simulink library "motohawk_engine_lib"  (Simulink 6.3)
undefined symbols (not defined in the file or in its folder): cast_val, IndPowerMax, InjSequence, lookup_group, MAF_Sensor_p, motohawk_tex, motohawk_vardec_config_group, motohawk_vardec_path, SampleTime, SparkSequence, SteadyStateECT, txtTitle, WarmUpTimeConst
libraries: MotoHawk_lib x234, motohawk_annotations_lib x22, motohawk_control_primitives_lib x20, motohawk_engine_lib x8, motohawk_control_primitives_lib_new x3
(part 1 of 7)
settings Model: Creator=Blake Suhre  LastModifiedBy=jason_tartt  StrictBusMsg=None

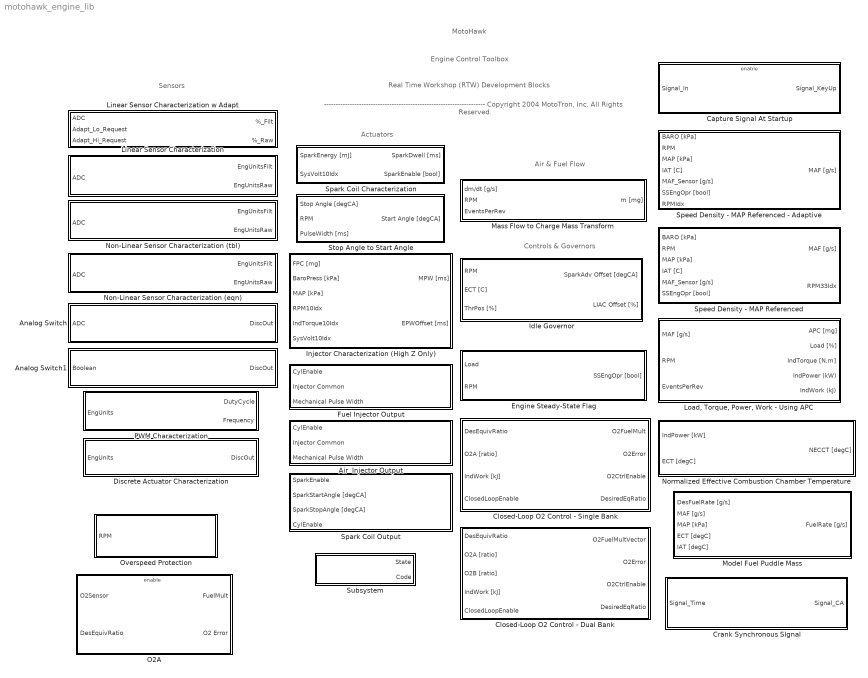
== system motohawk_engine_lib ==
  note: Sensors
  note: MotoHawk
  note: ---------------------------------------------------------------------
      | Copyright 2004 MotoTron, Inc.  All Rights Reserved.
  note: Real Time Workshop (RTW)
      | Development Blocks
  note: Engine Control Toolbox
  note: Actuators
  note: Air & Fuel Flow
  note: Controls & Governors
  Air  Injector Output : Subsystem  mask(Air Injector Hardware Interface){injector=1, offset=InjSequence(1)}
      mask prompts: offset "Angle Offset"
      mask help: Enter the air injector number.
      mask init:
      | lbl = sprintf('TRANSIENT\nAIR INJECTOR %d\n%d DEGREES', injector, offset);
      | 
      | blk = [gcb '/motohawk_injector'];
      | res = sprintf('AINJ%d', injector);
      | set_param(blk, 'text_resource', res);
      mask Display:
      | patch([0 0 1 1], [0 0.075 0.075 0], [230/255 0/255 0/255])
      | patch([0 0 1 1], [0.025 0.05 0.05 0.025], [150/255 0/255 0/255])
      | patch([0 0 1 1], [0 0.025 0.025 0], [0/255 0/255 0/255])
      | 
      | text(0.95, 0.5, lbl, 'horizontalAlignment', 'right');
  Analog Switch : Subsystem  mask{nam='PRNDL_D', prefix='PRNDL_D_', switchpoint=500, polarity=High-True, parent_group=lookup_group(gcb, 'Switches')}
      mask prompts: nam "Name"; switchpoint "Switch Point (ADC)"; parent_group "MotoTune Group"
      mask init:
      | lbl = ['Analog Switch: ' nam ' [bool]'];
      | group = [parent_group ' | ' nam];
      mask StyleString: edit,edit,edit,popup(High-True|Low-True),edit
      mask Display:
      | patch([0 0 1 1], [0 0.075 0.075 0], [230/255 0/255 0/255])
      | patch([0 0 1 1], [0.025 0.05 0.05 0.025], [150/255 0/255 0/255])
      | patch([0 0 1 1], [0 0.025 0.025 0], [0/255 0/255 0/255])
      | 
      | disp(lbl);
  Analog Switch1 : Subsystem  mask{nam='Digital', prefix=Digital_', polarity=High-True, parent_group='Switches'}
      mask prompts: nam "Name"; parent_group "MotoTune Group"
      mask init:
      | lbl = ['Digital Switch: ' nam ' [bool]'];
      | group = [parent_group ' | ' nam];
      mask StyleString: edit,edit,popup(High-True|Low-True),edit
      mask Display:
      | patch([0 0 1 1], [0 0.075 0.075 0], [230/255 0/255 0/255])
      | patch([0 0 1 1], [0.025 0.05 0.05 0.025], [150/255 0/255 0/255])
      | patch([0 0 1 1], [0 0.025 0.025 0], [0/255 0/255 0/255])
      | 
      | disp(lbl);
  Capture Signal At Startup : Subsystem  mask(Capture Signal At Startup){nam='Baro', count=5, units='kPa', grp='Engine Control | Run | Airflow'}
      mask prompts: nam "Signal Name"; count "Number Of Samples To Average"; grp "MotoTune GroupString Name"
      mask init:
      | lbl = sprintf('CAPTURE IN STALL\nAverage of\nfirst %d samples', count);
      mask Display:
      | patch([0 0 1 1], [0 0.075 0.075 0], [230/255 0/255 0/255])
      | patch([0 0 1 1], [0.025 0.05 0.05 0.025], [150/255 0/255 0/255])
      | patch([0 0 1 1], [0 0.025 0.025 0], [0/255 0/255 0/255])
      | 
      | disp(lbl);
  Closed-Loop O2 Control - Dual Bank : Subsystem
      mask Display:
      | patch([0 0 1 1], 0.5*[0 0.075 0.075 0], [230/255 0/255 0/255])
      | patch([0 0 1 1], 0.5*[0.025 0.05 0.05 0.025], [150/255 0/255 0/255])
      | patch([0 0 1 1], 0.5*[0 0.025 0.025 0], [0/255 0/255 0/255])
      | 
      | disp('DUAL BANK \nO2 CONTROL');
  Closed-Loop O2 Control - Single Bank : Subsystem
      mask Display:
      | patch([0 0 1 1], 0.5*[0 0.075 0.075 0], [230/255 0/255 0/255])
      | patch([0 0 1 1], 0.5*[0.025 0.05 0.05 0.025], [150/255 0/255 0/255])
      | patch([0 0 1 1], 0.5*[0 0.025 0.025 0], [0/255 0/255 0/255])
      | 
      | disp('SINGLE BANK \nO2 CONTROL');
  Crank Synchronous SIgnal : Subsystem
      mask Type: Crank Based Sensor Value
      mask Description: This subsystem averages input signal captured at 0 and 360 degrees.
      mask Display:
      | patch([0 0 1 1], [0 0.075 0.075 0], [230/255 0/255 0/255])
      | patch([0 0 1 1], [0.025 0.05 0.05 0.025], [150/255 0/255 0/255])
      | patch([0 0 1 1], [0 0.025 0.025 0], [0/255 0/255 0/255])
      | 
      | disp('CRANK SYNCHRONOUS \nSIGNAL')
  Discrete Actuator Characterization : Subsystem  mask(Discrete Actuator Characterization){prefix='MIL', nam='MIL', units='bool', parent_group='Actuators', polarity=High-True}
      mask prompts: nam "Name"; parent_group "MotoTune Group"
      mask help: Provides the ability to calibrate the polarity of the output digital state before it is applied to the digital output pin.
      mask init:
      | lbl = ['Discrete Characterization:  ' nam ];
      | group = [parent_group ' | ' nam];
      mask StyleString: edit,edit,edit,edit,popup(High-True|Low-True)
      mask Display:
      | patch([0 0 1 1], [0 0.075 0.075 0], [230/255 0/255 0/255])
      | patch([0 0 1 1], [0.025 0.05 0.05 0.025], [150/255 0/255 0/255])
      | patch([0 0 1 1], [0 0.025 0.025 0], [0/255 0/255 0/255])
      | 
      | disp(lbl);
  Engine Steady-State Flag : Subsystem  Description=|  mask(Steady-State Engine Operation){samp_time=SampleTime, group='Engine Control | States | States Config'}
      | /* Name: SSTorqueFilterConst Unit:sec ClassID:VAR StorageID:FLASH Access:RW4+RW3+NA2+NA1 TypeID:UINT2            
      |    Gain:0.001 Min:0.00 Max:65.54 Format:4.2 UpdateID:REMOTE Group:"Engine Control | States" Help:"First-order "  
      |    "filter time constant used to filter torque. This value must be less than SSTorqueTol from unfiltered torque "
      |    "before the steady-state flag can be enabled." VardecSig:6C */                                                
      |                                                                                                                  
      | /* Name: SSRPMFilterConst Unit:sec ClassID:VAR StorageID:FLASH Access:RW4+RW3+NA2+NA1 TypeID:UINT2               
      |    Gain:0.001 Min:0.00 Max:65.54 Format:4.2 UpdateID:REMOTE Group:"Engine Control | States" Help:"First-order "  
      |    "filter time constant used to filter torque. This value must be less than SSRPMTol from unfiltered torque "   
      |    "before the steady-state flag can be enabled." VardecSig:6C */                                                
      |                                                                                                                  
      | /* Name: SSTorqueTol Unit:N.m ClassID:VAR StorageID:FLASH Access:RW4+RW3+NA2+NA1 TypeID:UINT2 Gain:0.001         
      |    Min:0.00 Max:65.54 Format:4.2 UpdateID:REMOTE Group:"Engine Control | States" Help:"Tolerance within which "  
      |    "the difference between filtered and unfiltered torque must lie before the steady-state flag can be "         
      |    "enabled." VardecSig:6C */                                                                                    
      |                                                                                                                  
      | /* Name: SSRPMTol Unit:RPM ClassID:VAR StorageID:FLASH Access:RW4+RW3+NA2+NA1 TypeID:UINT2 Gain:0.01             
      |    Min:0.00 Max:655.35 Format:4.2 UpdateID:REMOTE Group:"Engine Control | States" Help:"Tolerance within which " 
      |    "the difference between filtered and unfiltered RPM must lie before the steady-state flag can be enabled."    
      |    VardecSig:6C */
      mask prompts: samp_time "Sample Time [s]:"; group "MotoTune Group String"
      mask help:
      | This block determines whether or not the engine has achieved steady-state operation. It accomplishes this by applying a first-order low-pass filter to the indicated torque and RPM inputs. The filetrcoeficeints are individually calibratable for each. Once both the filtered torque and RPM values are within the calibratable toleraance of the input values, engine operation is assumed to be steady-state.
      |
      | If 'Sample Time' is -1, then extra code and RAM will be generated to dynamically calculate dt.
      mask Display:
      | patch([0 0 1 1], [0 0.075 0.075 0], [230/255 0/255 0/255])
      | patch([0 0 1 1], [0.025 0.05 0.05 0.025], [150/255 0/255 0/255])
      | patch([0 0 1 1], [0 0.025 0.025 0], [0/255 0/255 0/255])
      | 
      | disp('ENGINE\nSTEADY-STATE\nDETERMINATION')
  Fuel Injector Output : Subsystem  mask(Fuel Injector Hardware Interface){injector=1, offset=InjSequence(1)}
      mask prompts: offset "Angle Offset"
      mask help: Enter the fuel injector number.
      mask init:
      | lbl = sprintf('TRANSIENT\nFUEL INJECTOR %d\n%d DEGREES', injector, offset);
      | 
      | blk = [gcb '/motohawk_injector'];
      | res = sprintf('FINJ%d', injector);
      | set_param(blk, 'text_resource', res);
      mask Display:
      | patch([0 0 1 1], [0 0.075 0.075 0], [230/255 0/255 0/255])
      | patch([0 0 1 1], [0.025 0.05 0.05 0.025], [150/255 0/255 0/255])
      | patch([0 0 1 1], [0 0.025 0.025 0], [0/255 0/255 0/255])
      | 
      | text(0.95, 0.5, lbl, 'horizontalAlignment', 'right');
  Idle Governor : Subsystem
      mask Display:
      | patch([0 0 1 1], 0.5*[0 0.075 0.075 0], [230/255 0/255 0/255])
      | patch([0 0 1 1], 0.5*[0.025 0.05 0.05 0.025], [150/255 0/255 0/255])
      | patch([0 0 1 1], 0.5*[0 0.025 0.025 0], [0/255 0/255 0/255])
      | 
      | disp('IDLE GOVERNOR');
  Injector Characterization (High Z Only) : Subsystem  Description=|
      | /* Name: InjGain Unit:ms/mg ClassID:VAR StorageID:FLASH Access:RW4+RW3+NA2+NA1 TypeID:UINT2 Gain:0.0001       
      |    Min:0.0000 Max:6.5500 Format:5.4 UpdateID:REMOTE Group:"Actuators | Injectors | Config" Help:"Gain valued "
      |    "used in the linear transformation of FPC to mechanical pulsewidth." VardecSig:6C */                       
      |                                                                                                               
      | /* Name: InjOfst Unit:ms ClassID:VAR StorageID:FLASH Access:RW4+RW3+NA2+NA1 TypeID:SINT2 Gain:0.0001          
      |    Min:-3.2768 Max:3.2767 Format:5.4 UpdateID:REMOTE Group:"Actuators | Injectors | Config" Help:"Offset "    
      |    "valued used in the linear transformation of FPC to mechanical pulsewidth." VardecSig:6C */                
      |                                                                                                               
      | /* Name: SysVolt10IdxArr Unit:volt ClassID:ORDARR StorageID:FLASH Access:RW4+RW3+NA2+NA1 TypeID:UINT1         
      |    Gain:0.1 Min:0.00 Max:25.50 Format:4.2 UpdateID:REMOTE OrdLen:10 Group:"Global Index Arrays | Voltage"     
      |    Help:"Ten breakpoint system voltage index array." VardecSig:6C */                                          
      |                                                                                                               
      | /* Name: InjTurnOnTbl Unit:ms ClassID:TBL StorageID:FLASH Access:RW4+RW3+NA2+NA1 TypeID:UINT2 Gain:0.001      
      |    Min:0.0000 Max:65.5350 Format:5.4 UpdateID:REMOTE OrdArr:SysVolt10IdxArr Group:"Actuators | Injectors"     
      |    Help:"Injector turn on time as a function of system voltage." VardecSig:6C */                              
      |                                                                                                               
      | /* Name: InjDeltaPress10IdxArr Unit:kPa ClassID:ORDARR StorageID:FLASH Access:RW4+RW3+NA2+NA1 TypeID:UINT2    
      |    Gain:0.1 Min:0.0 Max:6553.0 Format:5.1 UpdateID:REMOTE OrdLen:10 Group:"Actuators | Injectors" Help:"Ten " 
      |    "breakpoint fuel delta pressure index array." VardecSig:6C */                                              
      |                                                                                                               
      | /* Name: FueldPCompTbl Unit:kPa ClassID:TBL StorageID:FLASH Access:RW4+RW3+NA2+NA1 TypeID:UINT2 Gain:0.1      
      |    Min:0.0 Max:6553.0 Format:5.1 UpdateID:REMOTE OrdArr:InjDeltaPress10IdxArr Group:"Actuators | Injectors"   
      |    Help:"Injector delta pressure compensation table." VardecSig:6C */                                         
      |                                                                                                               
      | /* Name: InjTurnOffTbl Unit:ms ClassID:TBL StorageID:FLASH Access:RW4+RW3+NA2+NA1 TypeID:UINT2                
      |    Gain:0.01 Min:0.00 Max:655.00 Format:5.2 UpdateID:REMOTE OrdArr:InjDeltaPress10IdxArr Group:"Actuators | " 
      |    "Injectors" Help:"Injector turn off time table." VardecSig:6C */                                           
      |                                                                                                               
      | /* Name: InjMPW Unit:ms ClassID:VAR StorageID:RAM Access:RO4+RO3+NA2+NA1 TypeID:UINT2 Gain:0.01 Min:0.00      
      |    Max:655.35 Format:5.2 UpdateID:BACKGND Group:"Actuators | Injectors" Help:"Injector mechanical pulse "     
      |    "width." VardecSig:6C */                                                                                   
      |                                                                                                               
      | /* Name: InjEPW Unit:ms ClassID:VAR StorageID:RAM Access:RO4+RO3+NA2+NA1 TypeID:UINT2 Gain:0.01 Min:0.00      
      |    Max:655.35 Format:5.2 UpdateID:BACKGND Group:"Actuators | Injectors" Help:"Injector electrical pulse "     
      |    "width." VardecSig:6C */                                                                                   
      |                                                                                                               
      | /* Name: InjDeltaPress Unit:kPa ClassID:VAR StorageID:RAM Access:RO4+RO3+NA2+NA1 TypeID:UINT2 Gain:0.01       
      |    Min:0.00 Max:655.35 Format:5.2 UpdateID:BACKGND Group:"Actuators | Injectors" Help:"Delta pressure across "
      |    "the injector." VardecSig:6C */                                                                            
      | /* Name: FuelFlowCompMap Unit:mult ClassID:MAP StorageID:RAM Access:RO4+RO3+NA2+NA1 TypeID:UINT2              
      |    Gain:0.0001 Min:0.0000 Max:2.0000 Format:5.4 UpdateID:BACKGND XOrdArr:IndTorque10IdxArr YOrdArr:RPM10IdxArr
      |    Group:"Actuators | Injectors" Help:"Correction for injector fuel flow differences between injector test "  
      |    "bench and engine operating in the conditions. This map should only be calibrated after volumetric "       
      |    "efficiency has been calibrated to a reference airflow measurement device." VardecSig:6C */
      mask Description: Injector characterization block.
      mask Help: Converts the calculated fuel charge mass (FPC) value to the required electrical pulsewidth. Requires gain, offset, turn-on time vs. voltage, turn-off time vs. injector delta pressure and delta pressure pulsewidth compensation. A choice of five different injector delta pressure calculation methods are offered.
      mask Display:
      | patch([0 0 1 1], [0 0.075 0.075 0], [230/255 0/255 0/255])
      | patch([0 0 1 1], [0.025 0.05 0.05 0.025], [150/255 0/255 0/255])
      | patch([0 0 1 1], [0 0.025 0.025 0], [0/255 0/255 0/255])
      | 
      | disp('INJECTOR\nCHRZN.\n(High Z Only)')
  Linear Sensor Characterization : Subsystem  mask(Linear Sensor Characterization){nam='SysVolt', prefix='SysVolt_', units='Volts', inputunits=0, parent_group='Sensors | System Volts', samp_time=SampleTime}
      mask prompts: nam "Name"; units "Output Units"; inputunits "Input Units"; parent_group "MotoTune Group"; samp_time "Sample Time"
      mask help:
      | Converts from A/D Counts to Engineering Units, using a Gain and Offset.
      | Saturates the converted value around Min and Max values, and triggers a Fault when out of range.
      mask init:
      | lbl = ['Linear Sensor: ' nam ' [' units ']'];
      | group = [parent_group ' | ' nam];
      settings: RTWSystemCode=Function  RTWFcnNameOpts=Use subsystem name  RTWFileNameOpts=Use function name
      mask Display:
      | patch([0 0 1 1], [0 0.075 0.075 0], [230/255 0/255 0/255])
      | patch([0 0 1 1], [0.025 0.05 0.05 0.025], [150/255 0/255 0/255])
      | patch([0 0 1 1], [0 0.025 0.025 0], [0/255 0/255 0/255])
      | 
      | disp(lbl);
  Linear Sensor Characterization w Adapt : Subsystem  mask(Potentiometer Characterization with adapting endpoints.){nam='APP1', prefix='APP1', samp_time=.005, parent_group='Sensors | APP'}
      mask prompts: nam "Name"; samp_time "Sample Time"; parent_group "MotoTune Group"
      mask help:
      | This block transforms the input from a potentiometer into a percentage, refering to the percentage of travel within the scale.
      |
      | The endpoints of the scale will adapt based on the values that block sees on the input.
      mask init:
      | lbl = ['Linear Sensor: ' nam ' [%]'];
      | lbl2 = ['With Adaption'];
      | group = [parent_group ' | ' nam];
      | units = '%';
      mask Display:
      | patch([0 0 1 1], [0 0.075 0.075 0], [230/255 0/255 0/255])
      | patch([0 0 1 1], [0.025 0.05 0.05 0.025], [150/255 0/255 0/255])
      | patch([0 0 1 1], [0 0.025 0.025 0], [0/255 0/255 0/255])
      | 
      | 
      | 
      | text(0.6,0.60,lbl,'horizontalAlignment','center');
      | text(0.6,0.30,lbl2,'horizontalAlignment','center');
  "Load, Torque, Power, Work - Using APC" : Subsystem
      mask Display:
      | patch([0 0 1 1], 0.8*[0 0.075 0.075 0], [230/255 0/255 0/255])
      | patch([0 0 1 1], 0.8*[0.025 0.05 0.05 0.025], [150/255 0/255 0/255])
      | patch([0 0 1 1], 0.8*[0 0.025 0.025 0], [0/255 0/255 0/255])
      | 
      | disp('LOAD, TORQUE,\nPOWER, AND WORK\nCOMPUTATION\nUSING APC');
  Mass Flow to Charge Mass Transform : Subsystem
      mask Description: Converts mass flow rate to the equivalent per cylinder charge mass.
      mask Help:
      | Given the mass flow rate [g/s], RPM and the total number of combustion events per crankshaft revolution, this block calculates the equivalent charge mass ingested per cylinder.
      | 
      | Note: as an example, the number of cylinder events per revolution would be 2 for a four cylinder four-stroke engine and 4 for a four-cylinder two-stroke engine.
      mask Display:
      | patch([0 0 1 1], [0 0.075 0.075 0], [230/255 0/255 0/255])
      | patch([0 0 1 1], [0.025 0.05 0.05 0.025], [150/255 0/255 0/255])
      | patch([0 0 1 1], [0 0.025 0.025 0], [0/255 0/255 0/255])
      | 
      | disp('MASS FLOW\nTO CHARGE MASS\nTRANSFORM')
  Model Fuel Puddle Mass : Subsystem  mask{group_cal='Engine Control | Run | Fuel | Transient Fuel', group_dis='Engine Control | Run | Fuel | Transient Fuel'}
      mask prompts: group_cal "MotoTune Calibration Group String"; group_dis "MotoTune Display Group String"
      mask Display:
      | patch([0 0 1 1], 0.5*[0 0.075 0.075 0], [230/255 0/255 0/255])
      | patch([0 0 1 1], 0.5*[0.025 0.05 0.05 0.025], [150/255 0/255 0/255])
      | patch([0 0 1 1], 0.5*[0 0.025 0.025 0], [0/255 0/255 0/255])
      | 
      | disp('TAU-X\nTRANSIENT\nFUELING');
  Non-Linear Sensor Characterization (eqn) : Subsystem  mask(Non-Linear Sensor Characterization (eqn)){nam='MAF_Sensor', prefix='MAF_Sensor_', units='g/s', inputunits=0, parent_group=lookup_group(gcb, 'MAF_Sensor'), numcoef=MAF_Sensor_p, samp_time=SampleTime}
      mask prompts: nam "Name"; units "Output Units"; inputunits "Input Units"; parent_group "MotoTune Group"; numcoef "Number Of Coefficients"; samp_time "Sample Time"
      mask help:
      | Converts from A/D Counts to Engineering Units using a calibration polynomial.
      | Saturates the converted value around Min and Max values and triggers a Fault when out of range.
      mask init:
      | lbl = ['Non-Linear Sensor (eqn): ' nam ' [' units ']'];
      | group = [parent_group ' | ' nam];
      settings: RTWSystemCode=Function  RTWFcnNameOpts=Use subsystem name  RTWFileNameOpts=Use function name
      mask Display:
      | patch([0 0 1 1], [0 0.075 0.075 0], [230/255 0/255 0/255])
      | patch([0 0 1 1], [0.025 0.05 0.05 0.025], [150/255 0/255 0/255])
      | patch([0 0 1 1], [0 0.025 0.025 0], [0/255 0/255 0/255])
      | 
      | disp(lbl);
  Non-Linear Sensor Characterization (tbl) : Subsystem  mask(Non-Linear Sensor Characterization (tbl)){nam='MMA_Current', prefix='MMA_Current_', units='mA', inputunits='ADC', parent_group='Sensors', tblsize=20, samp_time=SampleTime}
      mask prompts: nam "Name"; units "Output Units"; inputunits "Input Units"; parent_group "MotoTune Group"; tblsize "Table Size"; samp_time "Sample Time"
      mask help:
      | Converts from A/D Counts to Engineering Units using a 1-D Table Lookup.
      | Saturates the converted value around Min and Max values and triggers a Fault when out of range.
      mask init:
      | lbl = ['Non-Linear Sensor (tbl): ' nam ' [' units ']'];
      | group = [parent_group ' | ' nam];
      settings: RTWSystemCode=Function  RTWFcnNameOpts=Use subsystem name  RTWFileNameOpts=Use function name
      mask Display:
      | patch([0 0 1 1], [0 0.075 0.075 0], [230/255 0/255 0/255])
      | patch([0 0 1 1], [0.025 0.05 0.05 0.025], [150/255 0/255 0/255])
      | patch([0 0 1 1], [0 0.025 0.025 0], [0/255 0/255 0/255])
      | 
      | disp(lbl);
  Normalized Effective Combustion Chamber Temperature : Subsystem  Description=|  mask(Steady-State Engine Operatio){}
      | /* Name: SSTorqueFilterConst Unit:sec ClassID:VAR StorageID:FLASH Access:RW4+RW3+NA2+NA1 TypeID:UINT2            
      |    Gain:0.001 Min:0.00 Max:65.54 Format:4.2 UpdateID:REMOTE Group:"Engine Control | States" Help:"First-order "  
      |    "filter time constant used to filter torque. This value must be less than SSTorqueTol from unfiltered torque "
      |    "before the steady-state flag can be enabled." VardecSig:6C */                                                
      |                                                                                                                  
      | /* Name: SSRPMFilterConst Unit:sec ClassID:VAR StorageID:FLASH Access:RW4+RW3+NA2+NA1 TypeID:UINT2               
      |    Gain:0.001 Min:0.00 Max:65.54 Format:4.2 UpdateID:REMOTE Group:"Engine Control | States" Help:"First-order "  
      |    "filter time constant used to filter torque. This value must be less than SSRPMTol from unfiltered torque "   
      |    "before the steady-state flag can be enabled." VardecSig:6C */                                                
      |                                                                                                                  
      | /* Name: SSTorqueTol Unit:N.m ClassID:VAR StorageID:FLASH Access:RW4+RW3+NA2+NA1 TypeID:UINT2 Gain:0.001         
      |    Min:0.00 Max:65.54 Format:4.2 UpdateID:REMOTE Group:"Engine Control | States" Help:"Tolerance within which "  
      |    "the difference between filtered and unfiltered torque must lie before the steady-state flag can be "         
      |    "enabled." VardecSig:6C */                                                                                    
      |                                                                                                                  
      | /* Name: SSRPMTol Unit:RPM ClassID:VAR StorageID:FLASH Access:RW4+RW3+NA2+NA1 TypeID:UINT2 Gain:0.01             
      |    Min:0.00 Max:655.35 Format:4.2 UpdateID:REMOTE Group:"Engine Control | States" Help:"Tolerance within which " 
      |    "the difference between filtered and unfiltered RPM must lie before the steady-state flag can be enabled."    
      |    VardecSig:6C */
      mask Display:
      | patch([0 0 1 1], [0 0.075 0.075 0], [230/255 0/255 0/255])
      | patch([0 0 1 1], [0.025 0.05 0.05 0.025], [150/255 0/255 0/255])
      | patch([0 0 1 1], [0 0.025 0.025 0], [0/255 0/255 0/255])
      | 
      | disp('COMBUSTION CHAMBER\nTEMPERATURE');
  O2A : Subsystem  TreatAsAtomicUnit=on  mask(Closed-Loop O2 Control){bank=A, display_group=lookup_group(gcb, 'O2Display'), cal_group=lookup_group(gcb, 'O2BankA')}
      mask prompts: display_group "MotoTune Display Group"; cal_group "MotoTune Calibration Group"
      mask StyleString: popup(A|B),edit,edit
      mask Display:
      | patch([0 0 1 1], 0.5*[0 0.075 0.075 0], [230/255 0/255 0/255])
      | patch([0 0 1 1], 0.5*[0.025 0.05 0.05 0.025], [150/255 0/255 0/255])
      | patch([0 0 1 1], 0.5*[0 0.025 0.025 0], [0/255 0/255 0/255])
      | 
      | disp(['O2 Control\nBank ' bank]);
  Overspeed Protection : Subsystem
      mask Description:
      | Block allows for three levels of overspeed rev limits, and will set three fault accordingly.
      | 
      | Soft Overspeed, Medium Overspeed, and Hard Overspeed.
      mask Display:
      | patch([0 0 1 1], 0.5*[0 0.075 0.075 0], [230/255 0/255 0/255])
      | patch([0 0 1 1], 0.5*[0.025 0.05 0.05 0.025], [150/255 0/255 0/255])
      | patch([0 0 1 1], 0.5*[0 0.025 0.025 0], [0/255 0/255 0/255])
      | 
      | disp('RPM LIMITER');
  PWM Characterization : Subsystem  mask(Linear Actuator Characterization){nam='LIAC', prefix='LIAC_', units='%', parent_group=motohawk_vardec_path(gcb)}
      mask prompts: nam "Name"; parent_group "MotoTune Group"
      mask help:
      | Scales the duty cycle of a PWM signal using a Gain and Offset with a calibratable PWM Frequency.
      | Saturates the converted value around Min and Max values, and converts the signal to the appropriate fixed-point format for use with motoHawk PWM blocks.
      mask init:
      | lbl = ['PWM Characterization: ' nam ];
      | group = [parent_group ' | ' nam];
      settings: RTWSystemCode=Function  RTWFcnNameOpts=Use subsystem name  RTWFileNameOpts=Use function name
      mask Display:
      | patch([0 0 1 1], [0 0.075 0.075 0], [230/255 0/255 0/255])
      | patch([0 0 1 1], [0.025 0.05 0.05 0.025], [150/255 0/255 0/255])
      | patch([0 0 1 1], [0 0.025 0.025 0], [0/255 0/255 0/255])
      | 
      | disp(lbl);
  Spark Coil Characterization : Subsystem  Description=|
      | /* Name: CoilDrvrDlyTime Unit:us ClassID:VAR StorageID:FLASH Access:RW4+RW3+NA2+NA1 TypeID:UINT2 Gain:0.1       
      |    Min:0.00 Max:6553.50 Format:6.2 UpdateID:REMOTE Group:"Actuators | Coils" Help:"Coil driver delay time "     
      |    "between initiation of the EST signal and the initiation of coil dwell." VardecSig:6C */                     
      |                                                                                                                 
      | /* Name: SysVolt10IdxArr Unit:volt ClassID:VAR StorageID:FLASH Access:RW4+RW3+NA2+NA1 TypeID:UINT1 Gain:0.1     
      |    Min:0.00 Max:25.50 Format:4.2 UpdateID:REMOTE Group:"Global Index Arrays | Voltage" Help:"Ten breakpoint "   
      |    "system voltage index array." VardecSig:6C */                                                                
      |                                                                                                                 
      | /* Name: SpkEnergy10IdxArr Unit:volt ClassID:VAR StorageID:FLASH Access:RW4+RW3+NA2+NA1 TypeID:UINT1            
      |    Gain:0.1 Min:0.00 Max:25.50 Format:4.2 UpdateID:REMOTE Group:"Actuators | Coils" Help:"Ten breakpoint spark "
      |    "energy index array." VardecSig:6C */                                                                        
      |                                                                                                                 
      | /* Name: CoilDwellMap Unit:ms ClassID:MAP StorageID:FLASH Access:RW4+RW3+NA2+NA1 TypeID:UINT2 Gain:0.01         
      |    Min:0.00 Max:655.35 Format:4.2 UpdateID:REMOTE XOrdArr:SpkEnergy10IdxArr YOrdArr:SysVolt10IdxArr             
      |    Group:"Actuators | Coils" Help:"Required coil dwell map as a function of system voltage and spark energy."   
      |    VardecSig:6C */
      mask Description: Coil characterization block.
      mask Help: Given the desired spark energy and system voltage, this block determines the required coil dwell period. Requires calibration of the dwell map and the delay time.
      mask Display:
      | patch([0 0 1 1], [0 0.075 0.075 0], [230/255 0/255 0/255])
      | patch([0 0 1 1], [0.025 0.05 0.05 0.025], [150/255 0/255 0/255])
      | patch([0 0 1 1], [0 0.025 0.025 0], [0/255 0/255 0/255])
      | 
      | disp('COIL\nCHRZN.')
  Spark Coil Output : Subsystem  mask(Spark Coil Hardware Interface){coil=1, offset=SparkSequence(1)}
      mask prompts: offset "Angle Offset"
      mask help: Enter the spark coil number (1-8)
      mask init:
      | lbl = sprintf('SPARK COIL %d\n%d DEGREES', coil, offset);
      | 
      | blk = [gcb '/motohawk_seq_out_est'];
      | set_param(blk, 'text_resource', sprintf('EST %d', coil));
      mask Display:
      | patch([0 0 1 1], [0 0.075 0.075 0], [230/255 0/255 0/255])
      | patch([0 0 1 1], [0.025 0.05 0.05 0.025], [150/255 0/255 0/255])
      | patch([0 0 1 1], [0 0.025 0.025 0], [0/255 0/255 0/255])
      | 
      | text(0.95, 0.5, lbl, 'horizontalAlignment', 'right');
  Speed Density - MAP Referenced : Subsystem  Description=|
      | /* Name: PortPressRatio20IdxArr Unit:unitless ClassID:ORDARR StorageID:FLASH Access:RW4+RW3+NA2+NA1              
      |    TypeID:UINT2 Gain:0.0001 Min:0.0000 Max:6.5535 Format:5.4 UpdateID:REMOTE OrdLen:20 Group:"Engine Control | " 
      |    "Run | Airflow" Help:"Port pressure ratio index array. Used for speed-density flow computations." VardecSig:6E
      |    */                                                                                                            
      |                                                                                                                  
      | /* Name: RPM20IdxArr Unit:RPM20IdxArr ClassID:ORDARR StorageID:FLASH Access:RW4+RW3+NA2+NA1                      
      |    TypeID:UINT2 Gain:0.1 Min:0.0 Max:6553.0 Format:5.1 UpdateID:REMOTE OrdLen:20 Group:"Global "                 
      |    "Index Arrays | RPM" Help:"20 breakpoint RPM index array." VardecSig:5E */                                    
      |                                                                                                                  
      | /* Name: VolEffMap Unit:Unitless ClassID:MAP StorageID:FLASH Access:RW4+RW3+NA2+NA1 TypeID:UINT2                 
      |    Gain:0.0001 Min:0.00 Max:6.55 Format:6.2 UpdateID:REMOTE XOrdArr:PortPressRatio20IdxArr                       
      |    YOrdArr:RPM20IdxArr Group:"Engine Control | Run | Airflow" Help:"Engine volumetric efficency "                
      |    "map." VardecSig:61 */                                                                                        
      |                                                                                                                  
      | /* Name: IAT10IdxArr Unit:C ClassID:ORDARR StorageID:FLASH Access:RW4+RW3+NA2+NA1                                
      |    TypeID:SINT2 Gain:0.01 Min:-327.6800 Max:327.6700 Format:5.4 UpdateID:REMOTE OrdLen:10                        
      |    Group:"Engine Control | Run | Airflow" Help:"10 breakpoint intake air temperture index "                      
      |    "array." VardecSig:5C */                                                                                      
      |                                                                                                                  
      | /* Name: VETempCorrTbl ClassID:TBL StorageID:FLASH Access:RW4+RW3+NA2+NA1 TypeID:UINT2 Gain:0.0001 Min:0.00      
      |    Max:6.55 Format:4.2 UpdateID:REMOTE OrdArr:IAT10IdxArr Group:"Engine Control | Run | Airflow"                 
      |    Help:"Volumetric efficiency temperature correction table." VardecSig:6C */                                    
      |                                                                                                                  
      | /* Name: BaroPress10IdxArr Unit:C ClassID:ORDARR StorageID:FLASH Access:RW4+RW3+NA2+NA1                          
      |    TypeID:UINT2 Gain:0.01 Min:0.0000 Max:655.3500 Format:5.4 UpdateID:REMOTE OrdLen:10                           
      |    Group:"Engine Control | Run | Airflow" Help:"10 breakpoint barometric pressure index "                        
      |    "array." VardecSig:5C */                                                                                      
      |                                                                                                                  
      | /* Name: VEBaroCorrTbl ClassID:TBL StorageID:FLASH Access:RW4+RW3+NA2+NA1 TypeID:UINT2 Gain:0.0001 Min:0.00      
      |    Max:6.55 Format:4.2 UpdateID:REMOTE OrdArr:BaroPress10IdxArr Group:"Engine Control | Run | Airflow"           
      |    Help:"Volumetric efficiency barometric pressure correction table." VardecSig:6C */                            
      |                                                                                                                  
      | /* Name: CylSweptVol Unit:cm^3 ClassID:VAR StorageID:FLASH Access:RW4+RW3+NA2+NA1 TypeID:UINT2 Gain:0.1          
      |    Min:0.0 Max:6553.0 Format:5.1 UpdateID:REMOTE Group:"Engine Control | Run | Airflow" Help:"Cylinder swept "   
      |    "volume." VardecSig:6C */                                                                                     
      |                                                                                                                  
      | /* Name: MAFPort Unit:g/s ClassID:VAR StorageID:RAM Access:RO4+RO3+NA2+NA1 TypeID:UINT2 Gain:0.01                
      |    Min:0.00 Max:655.00 Format:5.2 UpdateID:BACKGND Group:"Engine Control | Run | Airflow" Help:"Total "          
      |    "ingested cylinder charge mass flow rate. The sum of all port flows. This values includes any EGR and "       
      |    "Purge mass flows." VardecSig:6A */                                                                           
      |                                                                                                                  
      | /* Name: CombEventsPerRev ClassID:VAR StorageID:FLASH Access:RW4+RW3+NA2+NA1 TypeID:UINT1 Gain:0.5 Min:0.5       
      |    Max:127.0 Format:4.1 UpdateID:REMOTE Group:"Engine Control | Run | Airflow" Help:"Number of conbustion "      
      |    "events per engine revolution. For example, for a four-stroke, eight cylinder engine the value would be 4."   
      |    VardecSig:6C */
      mask Description: Calculates air mass flow rate per cylinder. The estimated mass flow rate is that of the entire mixture: air, EGR and purge.
      mask Help: Given calibrations for the volumetric efficiency map, cylinder swept volume [cm3] and the VE temperature and pressure correction tables, the block calculates the air mass flow rate [g/s] per cylinder, given the barometric and manifold pressures [kPa], the manifold air temperature [C] and RPM.
      mask Display:
      | patch([0 0 1 1], 0.5*[0 0.075 0.075 0], [230/255 0/255 0/255])
      | patch([0 0 1 1], 0.5*[0.025 0.05 0.05 0.025], [150/255 0/255 0/255])
      | patch([0 0 1 1], 0.5*[0 0.025 0.025 0], [0/255 0/255 0/255])
      | 
      | disp('MAP-REFERENCED\nSPEED-DENSITY\nCOMPUTATION');
  Speed Density - MAP Referenced - Adaptive : Subsystem  Description=|
      | /* Name: PortPressRatio20IdxArr Unit:unitless ClassID:ORDARR StorageID:FLASH Access:RW4+RW3+NA2+NA1              
      |    TypeID:UINT2 Gain:0.0001 Min:0.0000 Max:6.5535 Format:5.4 UpdateID:REMOTE OrdLen:20 Group:"Engine Control | " 
      |    "Run | Airflow" Help:"Port pressure ratio index array. Used for speed-density flow computations." VardecSig:6E
      |    */                                                                                                            
      |                                                                                                                  
      | /* Name: RPM20IdxArr Unit:RPM20IdxArr ClassID:ORDARR StorageID:FLASH Access:RW4+RW3+NA2+NA1                      
      |    TypeID:UINT2 Gain:0.1 Min:0.0 Max:6553.0 Format:5.1 UpdateID:REMOTE OrdLen:20 Group:"Global "                 
      |    "Index Arrays | RPM" Help:"20 breakpoint RPM index array." VardecSig:5E */                                    
      |                                                                                                                  
      | /* Name: VolEffMap Unit:Unitless ClassID:MAP StorageID:FLASH Access:RW4+RW3+NA2+NA1 TypeID:UINT2                 
      |    Gain:0.0001 Min:0.00 Max:6.55 Format:6.2 UpdateID:REMOTE XOrdArr:PortPressRatio20IdxArr                       
      |    YOrdArr:RPM20IdxArr Group:"Engine Control | Run | Airflow" Help:"Engine volumetric efficency "                
      |    "map." VardecSig:61 */                                                                                        
      |                                                                                                                  
      | /* Name: IAT10IdxArr Unit:C ClassID:ORDARR StorageID:FLASH Access:RW4+RW3+NA2+NA1                                
      |    TypeID:SINT2 Gain:0.01 Min:-327.6800 Max:327.6700 Format:5.4 UpdateID:REMOTE OrdLen:10                        
      |    Group:"Engine Control | Run | Airflow" Help:"10 breakpoint intake air temperture index "                      
      |    "array." VardecSig:5C */                                                                                      
      |                                                                                                                  
      | /* Name: VETempCorrTbl ClassID:TBL StorageID:FLASH Access:RW4+RW3+NA2+NA1 TypeID:UINT2 Gain:0.0001 Min:0.00      
      |    Max:6.55 Format:4.2 UpdateID:REMOTE OrdArr:IAT10IdxArr Group:"Engine Control | Run | Airflow"                 
      |    Help:"Volumetric efficiency temperature correction table." VardecSig:6C */                                    
      |                                                                                                                  
      | /* Name: BaroPress10IdxArr Unit:C ClassID:ORDARR StorageID:FLASH Access:RW4+RW3+NA2+NA1                          
      |    TypeID:UINT2 Gain:0.01 Min:0.0000 Max:655.3500 Format:5.4 UpdateID:REMOTE OrdLen:10                           
      |    Group:"Engine Control | Run | Airflow" Help:"10 breakpoint barometric pressure index "                        
      |    "array." VardecSig:5C */                                                                                      
      |                                                                                                                  
      | /* Name: VEBaroCorrTbl ClassID:TBL StorageID:FLASH Access:RW4+RW3+NA2+NA1 TypeID:UINT2 Gain:0.0001 Min:0.00      
      |    Max:6.55 Format:4.2 UpdateID:REMOTE OrdArr:BaroPress10IdxArr Group:"Engine Control | Run | Airflow"           
      |    Help:"Volumetric efficiency barometric pressure correction table." VardecSig:6C */                            
      |                                                                                                                  
      | /* Name: CylSweptVol Unit:cm^3 ClassID:VAR StorageID:FLASH Access:RW4+RW3+NA2+NA1 TypeID:UINT2 Gain:0.1          
      |    Min:0.0 Max:6553.0 Format:5.1 UpdateID:REMOTE Group:"Engine Control | Run | Airflow" Help:"Cylinder swept "   
      |    "volume." VardecSig:6C */                                                                                     
      |                                                                                                                  
      | /* Name: MAFPort Unit:g/s ClassID:VAR StorageID:RAM Access:RO4+RO3+NA2+NA1 TypeID:UINT2 Gain:0.01                
      |    Min:0.00 Max:655.00 Format:5.2 UpdateID:BACKGND Group:"Engine Control | Run | Airflow" Help:"Total "          
      |    "ingested cylinder charge mass flow rate. The sum of all port flows. This values includes any EGR and "       
      |    "Purge mass flows." VardecSig:6A */                                                                           
      |                                                                                                                  
      | /* Name: CombEventsPerRev ClassID:VAR StorageID:FLASH Access:RW4+RW3+NA2+NA1 TypeID:UINT1 Gain:0.5 Min:0.5       
      |    Max:127.0 Format:4.1 UpdateID:REMOTE Group:"Engine Control | Run | Airflow" Help:"Number of conbustion "      
      |    "events per engine revolution. For example, for a four-stroke, eight cylinder engine the value would be 4."   
      |    VardecSig:6C */
      mask Description: Calculates air mass flow rate per cylinder. The estimated mass flow rate is that of the entire mixture: air, EGR and purge.
      mask Help: Given calibrations for the volumetric efficiency map, cylinder swept volume [cm3] and the VE temperature and pressure correction tables, the block calculates the air mass flow rate [g/s] per cylinder, given the barometric and manifold pressures [kPa], the manifold air temperature [C] and RPM.
      mask Display:
      | patch([0 0 1 1], 0.5*[0 0.075 0.075 0], [230/255 0/255 0/255])
      | patch([0 0 1 1], 0.5*[0.025 0.05 0.05 0.025], [150/255 0/255 0/255])
      | patch([0 0 1 1], 0.5*[0 0.025 0.025 0], [0/255 0/255 0/255])
      | 
      | disp('MAP-REFERENCED\nSPEED-DENSITY\nCOMPUTATION\n(adaptive)');
  Stop Angle to Start Angle : Subsystem  Description=|
      | /* Name: CoilDrvrDlyTime Unit:us ClassID:VAR StorageID:FLASH Access:RW4+RW3+NA2+NA1 TypeID:UINT2 Gain:0.1       
      |    Min:0.00 Max:6553.50 Format:6.2 UpdateID:REMOTE Group:"Actuators | Coils" Help:"Coil driver delay time "     
      |    "between initiation of the EST signal and the initiation of coil dwell." VardecSig:6C */                     
      |                                                                                                                 
      | /* Name: SysVolt10IdxArr Unit:volt ClassID:VAR StorageID:FLASH Access:RW4+RW3+NA2+NA1 TypeID:UINT1 Gain:0.1     
      |    Min:0.00 Max:25.50 Format:4.2 UpdateID:REMOTE Group:"Global Index Arrays | Voltage" Help:"Ten breakpoint "   
      |    "system voltage index array." VardecSig:6C */                                                                
      |                                                                                                                 
      | /* Name: SpkEnergy10IdxArr Unit:volt ClassID:VAR StorageID:FLASH Access:RW4+RW3+NA2+NA1 TypeID:UINT1            
      |    Gain:0.1 Min:0.00 Max:25.50 Format:4.2 UpdateID:REMOTE Group:"Actuators | Coils" Help:"Ten breakpoint spark "
      |    "energy index array." VardecSig:6C */                                                                        
      |                                                                                                                 
      | /* Name: CoilDwellMap Unit:ms ClassID:MAP StorageID:FLASH Access:RW4+RW3+NA2+NA1 TypeID:UINT2 Gain:0.01         
      |    Min:0.00 Max:655.35 Format:4.2 UpdateID:REMOTE XOrdArr:SpkEnergy10IdxArr YOrdArr:SysVolt10IdxArr             
      |    Group:"Actuators | Coils" Help:"Required coil dwell map as a function of system voltage and spark energy."   
      |    VardecSig:6C */
      mask Type: Stop Angle to Start Angle
      mask Description: Stop Angle to Start Angle calculation.  Subtracts the duration of a Pulse Width in the angle domain from a given Stop Angle.
      mask Display:
      | patch([0 0 1 1], [0 0.075 0.075 0], [230/255 0/255 0/255])
      | patch([0 0 1 1], [0.025 0.05 0.05 0.025], [150/255 0/255 0/255])
      | patch([0 0 1 1], [0 0.025 0.025 0], [0/255 0/255 0/255])
  Subsystem : Subsystem  mask{fltnam='FaultName'}
      mask prompts: fltnam "Fault Name"
      mask Display:
      | patch([0 0 1 1], 0.5*[0 0.075 0.075 0], [230/255 0/255 0/255])
      | patch([0 0 1 1], 0.5*[0.025 0.05 0.05 0.025], [150/255 0/255 0/255])
      | patch([0 0 1 1], 0.5*[0 0.025 0.025 0], [0/255 0/255 0/255])
      | 
      | disp(['Fault Code\n' fltnam]);

== system motohawk_engine_lib/Air  Injector Output ==
  CylEnable : Inport
  Injector Common : Inport  Port=2
  Mechanical Pulse Width : Inport  Port=3
  Bus Selector : BusSelector  OutputSignals=Enable,SOI,PeakEPW,InjEPWOffset,EOI,MakeupMin
  Data Type Conversion{1..6} (6 alike) : DataTypeConversion  SaturateOnIntegerOverflow=on  RndMeth=Zero
  Gain{1,3..4,6} (4 alike) : Gain  Gain=1000  SaturateOnIntegerOverflow=on
  Gain2 : Gain  Gain=16  SaturateOnIntegerOverflow=on
  Gain5 : Gain  Gain=16  SaturateOnIntegerOverflow=on
  Logical Operator : Logic  AllPortsSameDT=off
  motohawk_injector : MotoHawk_lib/Advanced Digital I//O/motohawk_injector  text_resource=AINJ1  code_resource=RES_INJ1D  val_resource=-1  target=ECU555_80  resource_enum_str=(None)=-1,FINJ1=12,FINJ2=13,FINJ3=14,FINJ4=15,FINJ5=16,FINJ6=17,FINJ7=18,AINJ1=18,FINJ8=19,AINJ2=19,FINJ9=20,AINJ3=20,FINJ10=21,AINJ4=21,FINJ11=22,AINJ5=22,FINJ12=23,AINJ6=23  behavior=Transient  update_mode=OS  granularity=Fine  angle_offset=offset  min_eoi_soi_angle=90  use_vardec=off  nam='INJ'  read_level=1  write_level=1  group='System | I/O Pins | Outputs Config'
  wires:
  Data Type Conversion5/1 -> motohawk_injector/6
  Data Type Conversion2/1 -> motohawk_injector/3
  Data Type Conversion6/1 -> motohawk_injector/7
  Data Type Conversion3/1 -> motohawk_injector/5
  Data Type Conversion4/1 -> motohawk_injector/4
  Data Type Conversion1/1 -> motohawk_injector/2
  Gain6/1 -> Data Type Conversion6/1
  Gain5/1 -> Data Type Conversion5/1
  Injector Common/1 -> Bus Selector/1
  Gain4/1 -> Data Type Conversion4/1
  Gain1/1 -> Data Type Conversion2/1
  Gain2/1 -> Data Type Conversion1/1
  Bus Selector/4 -> Gain3/1  "<InjEPWOffset>"
  Gain3/1 -> Data Type Conversion3/1
  Bus Selector/6 -> Gain6/1  "<MakeupMin>"
  Bus Selector/3 -> Gain4/1  "<PeakEPW>"
  Mechanical Pulse Width/1 -> Gain1/1
  Bus Selector/5 -> Gain5/1  "<EOI>"
  Bus Selector/2 -> Gain2/1  "<SOI>"
  Bus Selector/1 -> Logical Operator/2  "<Enable>"
  CylEnable/1 -> Logical Operator/1
  Logical Operator/1 -> motohawk_injector/1
